simulink model "Q1"  (R2017a)
settings: Solver=VariableStepAuto  StartTime=0.0  StopTime=200  RelTol=1e-3
undefined symbols (not defined in the file or in its folder): m, n
settings Model: Creator=hp  LastModifiedBy=hp
settings DataIOCC: SaveOutput=off  SaveTime=off

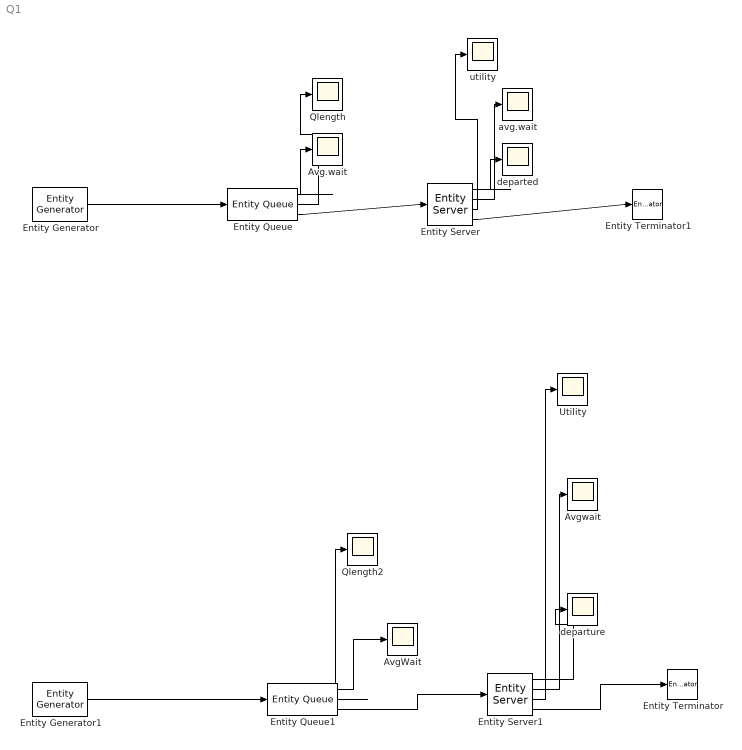
== system Q1 ==
  Avg.wait : Scope
  AvgWait : Scope
  Avgwait : Scope
  Entity Generator : EntityGenerator  OutputPortMessageModes=m  TimeSource=MATLAB action  IntergenerationTimeAction=dt = exprnd(0.3);  EntityType=Structured  EntityTypeName=Entity
  Entity Generator1 : EntityGenerator  OutputPortMessageModes=m  TimeSource=MATLAB action  IntergenerationTimeAction=dt = exprnd(0.3);  EntityType=Structured  EntityTypeName=Entity
  Entity Queue : EntityQueue  InputPortMessageModes=m  OutputPortMessageModes=n,n,m  Capacity=inf  QueueType=LIFO  AverageWait=on  AverageQueueLength=on
      settings: OutputPortMap=o2,o3,o5
  Entity Queue1 : EntityQueue  InputPortMessageModes=m  OutputPortMessageModes=n,n,m  Capacity=inf  AverageWait=on  AverageQueueLength=on
      settings: OutputPortMap=o2,o3,o5
  Entity Server : EntityServer  InputPortMessageModes=m  OutputPortMessageModes=n,n,n,m  Capacity=1  ServiceTimeSource=MATLAB action  ServiceTimeAction=|  NumberEntitiesDeparted=on  AverageWait=on  Utilization=on
      | function dt = f()
      |     coder.extrinsic('get_param');
      |     t = 1 + (199).*rand(1,1);;
      |     if t < 100
      |         dt = exprnd(2);
      |     else
      |         dt = normrnd(3, 0.1);
      |     end
      | end
      | 
      | dt = f();
      settings: OutputPortMap=o0,o4,o5,o9
  Entity Server1 : EntityServer  InputPortMessageModes=m  OutputPortMessageModes=n,n,n,m  Capacity=1  ServiceTimeSource=MATLAB action  ServiceTimeAction=|  NumberEntitiesDeparted=on  AverageWait=on  Utilization=on
      | function dt = f()
      |     t = (200).*rand(1,1);
      |     if t < 100
      |         dt = exprnd(2);
      |     else
      |         dt = normrnd(3, 0.1);
      |     end
      | end
      | 
      | dt = f();
      settings: OutputPortMap=o0,o4,o5,o9
  Entity Terminator : EntityTerminator  InputPortMessageModes=m
  Entity Terminator1 : EntityTerminator  InputPortMessageModes=m
  Qlength : Scope
  Qlength2 : Scope
  "Utility " : Scope
  avg.wait : Scope
  "departed " : Scope
  departure : Scope
  utility : Scope
  wires:
  Entity Generator/1 -> Entity Queue/1
  Entity Queue/3 -> Entity Server/1
  Entity Queue/1 -> Avg.wait/1
  Entity Queue/2 -> Qlength/1
  Entity Server/3 -> utility/1
  Entity Server/2 -> avg.wait/1
  Entity Server/1 -> "departed "/1
  Entity Generator1/1 -> Entity Queue1/1
  Entity Queue1/3 -> Entity Server1/1
  Entity Server1/3 -> "Utility "/1
  Entity Server1/2 -> Avgwait/1
  Entity Server1/1 -> departure/1
  Entity Queue1/2 -> Qlength2/1
  Entity Queue1/1 -> AvgWait/1
  Entity Server1/4 -> Entity Terminator/1
  Entity Server/4 -> Entity Terminator1/1
